simulink model "QAM_Show"  (R2014a)
settings: Solver=ode45  StartTime=0.0  StopTime=10  RelTol=1e-3
libraries: commrandsrc2 x7, commdigbbndam3 x7
CloseFcn:
  | clear phnoiseSigsOut
  | 
  | % Close BER figure, if it exists
  | if exist('hPhaseNoise256QAM')  % figure has been created
  |     if ishandle(hPhaseNoise256QAM)  % figure still exists
  |         close(hPhaseNoise256QAM)
  |     end
  |     clear hPhaseNoise256QAM
  | end
Description:
  | Phase Noise Effects in 256-QAM
  | 
  | This model shows the effect of a receiver's phase noise on 256-ary quadrature amplitude modulation (QAM).
settings Model: ExtModeAutoUpdateStatusClock=off  Creator=The MathWorks Inc.  LastModifiedBy=okuu
settings SolverCC: InsertRTBMode=Auto
settings DataIOCC: SignalLoggingSaveFormat=ModelDataLogs  SaveOutput=off  SaveTime=off  SignalLoggingName=phnoiseSigsOut
settings OptimizationCC: BlockReduction=off  BooleanDataType=off  ExpressionDepthLimit=2147483647  InitFltsAndDblsToZero=on  EfficientMapNaN2IntZero=off  BufferReusableBoundary=off
settings DebuggingCC: SaveWithParameterizedLinksMsg=none  UnderspecifiedInitializationDetection=Classic  CheckExecutionContextPreStartOutputMsg=on  CheckExecutionContextRuntimeOutputMsg=on  SignalResolutionControl=TryResolveAllWithWarning  SolverPrmCheckMsg=none  InheritedTsInSrcMsg=none  MultiTaskDSMMsg=warning  MultiTaskCondExecSysMsg=none  SigSpecEnsureSampleTimeMsg=none  ParameterPrecisionLossMsg=none  FcnCallInpInsideContextMsg=UseLocalSettings  BusObjectLabelMismatch=none  StateNameClashWarn=warning
settings HardwareCC: TargetUnknown=on
settings ModelReferenceCC: UpdateModelReferenceTargets=IfOutOfDate
settings RTWCC: IncludeERTFirstTime=on
settings GRTTargetCC: TargetFcnLib=ansi_tfl_tmw.mat  CombineOutputUpdateFcns=off  GRTInterface=on

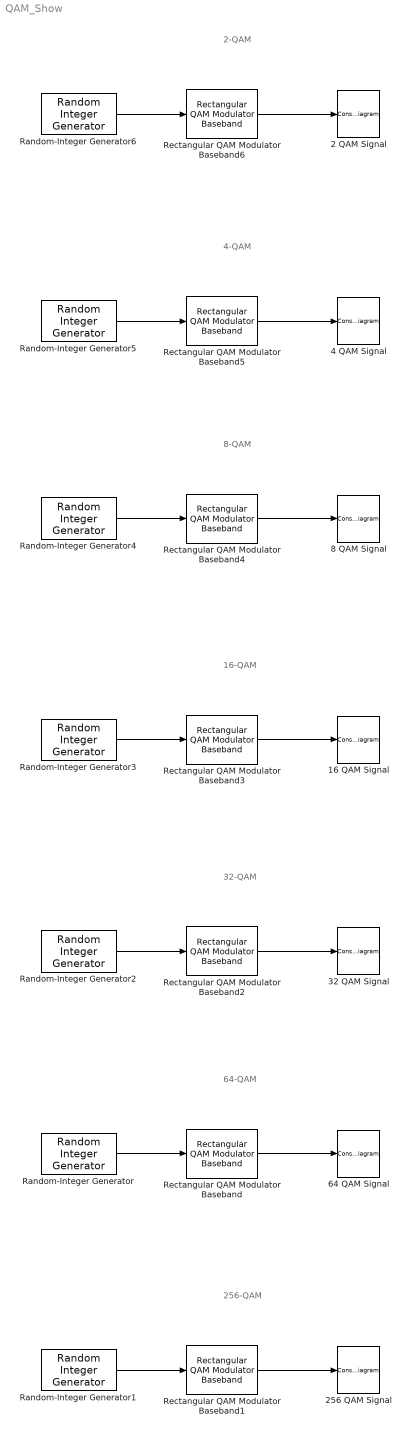
== system QAM_Show ==
  note: 64-QAM
  note: 256-QAM
  note: 32-QAM
  note: 16-QAM
  note: 8-QAM
  note: 4-QAM
  note: 2-QAM
  16 QAM Signal : ConstellationDiagram  Tag=ScatterPlot
  2 QAM Signal : ConstellationDiagram  Tag=ScatterPlot
  256 QAM Signal : ConstellationDiagram  Tag=ScatterPlot
  32 QAM Signal : ConstellationDiagram  Tag=ScatterPlot
  4 QAM Signal : ConstellationDiagram  Tag=ScatterPlot
  64 QAM Signal : ConstellationDiagram  Tag=ScatterPlot
  8 QAM Signal : ConstellationDiagram  Tag=ScatterPlot
  Random-Integer Generator : commrandsrc2/Random Integer Generator  mul=64  seed=12345  Ts=.001  frameBased=on  sampPerFrame=500  orient=off  outDataType=uint8
  Random-Integer Generator1 : commrandsrc2/Random Integer Generator  mul=256  seed=12345  Ts=.001  frameBased=on  sampPerFrame=500  orient=off  outDataType=uint8
  Random-Integer Generator2 : commrandsrc2/Random Integer Generator  mul=32  seed=12345  Ts=.001  frameBased=on  sampPerFrame=500  orient=off  outDataType=uint8
  Random-Integer Generator3 : commrandsrc2/Random Integer Generator  mul=16  seed=12345  Ts=.001  frameBased=on  sampPerFrame=500  orient=off  outDataType=uint8
  Random-Integer Generator4 : commrandsrc2/Random Integer Generator  mul=8  seed=12345  Ts=.001  frameBased=on  sampPerFrame=500  orient=off  outDataType=uint8
  Random-Integer Generator5 : commrandsrc2/Random Integer Generator  mul=4  seed=12345  Ts=.001  frameBased=on  sampPerFrame=500  orient=off  outDataType=uint8
  Random-Integer Generator6 : commrandsrc2/Random Integer Generator  mul=2  seed=12345  Ts=.001  frameBased=on  sampPerFrame=500  orient=off  outDataType=uint8
  Rectangular QAM Modulator Baseband : commdigbbndam3/Rectangular QAM Modulator Baseband  M=64  InType=Integer  Enc=Gray  Mapping=[0:15]  PowType=Average Power  MinDist=2  AvgPow=1  PeakPow=1  Ph=0  outDtype=single  outWordLen=16  outUDDataType=sfix(16)  outFracLenMode=Best precision  outFracLen=15
  Rectangular QAM Modulator Baseband1 : commdigbbndam3/Rectangular QAM Modulator Baseband  M=256  InType=Integer  Enc=Gray  Mapping=[0:15]  PowType=Average Power  MinDist=2  AvgPow=1  PeakPow=1  Ph=0  outDtype=single  outWordLen=16  outUDDataType=sfix(16)  outFracLenMode=Best precision  outFracLen=15
  Rectangular QAM Modulator Baseband2 : commdigbbndam3/Rectangular QAM Modulator Baseband  M=32  InType=Integer  Enc=Gray  Mapping=[0:15]  PowType=Average Power  MinDist=2  AvgPow=1  PeakPow=1  Ph=0  outDtype=single  outWordLen=16  outUDDataType=sfix(16)  outFracLenMode=Best precision  outFracLen=15
  Rectangular QAM Modulator Baseband3 : commdigbbndam3/Rectangular QAM Modulator Baseband  M=16  InType=Integer  Enc=Gray  Mapping=[0:15]  PowType=Average Power  MinDist=2  AvgPow=1  PeakPow=1  Ph=0  outDtype=single  outWordLen=16  outUDDataType=sfix(16)  outFracLenMode=Best precision  outFracLen=15
  Rectangular QAM Modulator Baseband4 : commdigbbndam3/Rectangular QAM Modulator Baseband  M=8  InType=Integer  Enc=Gray  Mapping=[0:15]  PowType=Average Power  MinDist=2  AvgPow=1  PeakPow=1  Ph=0  outDtype=single  outWordLen=16  outUDDataType=sfix(16)  outFracLenMode=Best precision  outFracLen=15
  Rectangular QAM Modulator Baseband5 : commdigbbndam3/Rectangular QAM Modulator Baseband  M=4  InType=Integer  Enc=Gray  Mapping=[0:15]  PowType=Average Power  MinDist=2  AvgPow=1  PeakPow=1  Ph=0  outDtype=single  outWordLen=16  outUDDataType=sfix(16)  outFracLenMode=Best precision  outFracLen=15
  Rectangular QAM Modulator Baseband6 : commdigbbndam3/Rectangular QAM Modulator Baseband  M=2  InType=Integer  Enc=Gray  Mapping=[0:15]  PowType=Average Power  MinDist=2  AvgPow=1  PeakPow=1  Ph=0  outDtype=single  outWordLen=16  outUDDataType=sfix(16)  outFracLenMode=Best precision  outFracLen=15
  wires:
  Random-Integer Generator/1 -> Rectangular QAM Modulator Baseband/1
  Rectangular QAM Modulator Baseband/1 -> 64 QAM Signal/1
  Random-Integer Generator1/1 -> Rectangular QAM Modulator Baseband1/1
  Rectangular QAM Modulator Baseband1/1 -> 256 QAM Signal/1
  Random-Integer Generator2/1 -> Rectangular QAM Modulator Baseband2/1
  Rectangular QAM Modulator Baseband2/1 -> 32 QAM Signal/1
  Random-Integer Generator3/1 -> Rectangular QAM Modulator Baseband3/1
  Rectangular QAM Modulator Baseband3/1 -> 16 QAM Signal/1
  Random-Integer Generator4/1 -> Rectangular QAM Modulator Baseband4/1
  Rectangular QAM Modulator Baseband4/1 -> 8 QAM Signal/1
  Random-Integer Generator5/1 -> Rectangular QAM Modulator Baseband5/1
  Rectangular QAM Modulator Baseband5/1 -> 4 QAM Signal/1
  Random-Integer Generator6/1 -> Rectangular QAM Modulator Baseband6/1
  Rectangular QAM Modulator Baseband6/1 -> 2 QAM Signal/1
